simulink model "lab_single_phse_inv_1"  (R2019a)
settings: Solver=VariableStepAuto  StartTime=0.0  StopTime=0.1  RelTol=1e-3
libraries: powerlib x12, simulink x1
settings Model: Creator=Manish  LastModifiedBy=Manish

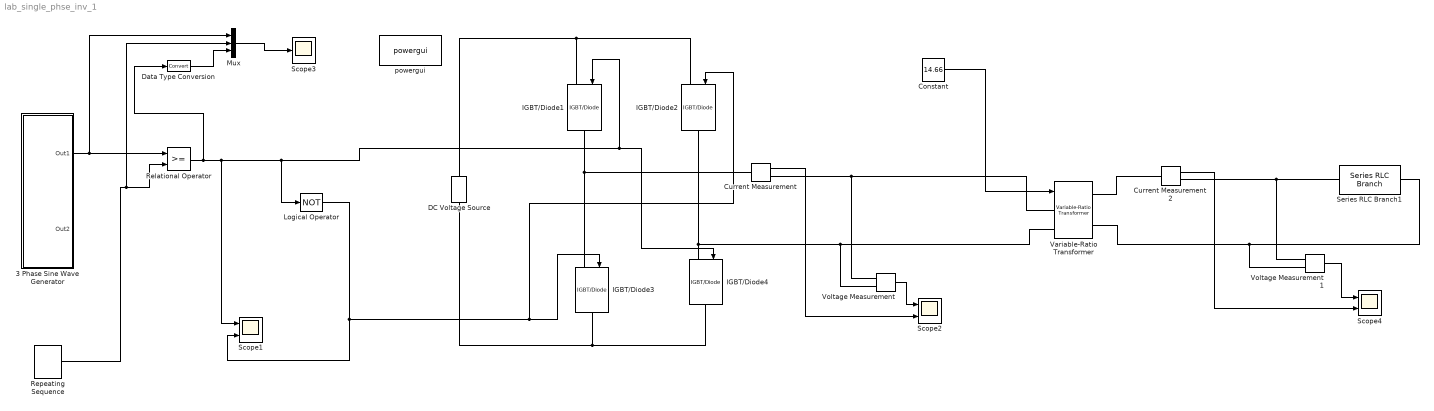
== system lab_single_phse_inv_1 ==
  3 Phase Sine Wave Generator : Subsystem
  Constant : Constant  Value=14.66
  Current Measurement : powerlib/Measurements/Current Measurement  PhasorSimulation=off  OutputType=Complex  PSBequivalent=0
  Current Measurement2 : powerlib/Measurements/Current Measurement  PhasorSimulation=off  OutputType=Complex  PSBequivalent=0
  DC Voltage Source : powerlib/Electrical Sources/DC Voltage Source  Amplitude=24  Measurements=None
  Data Type Conversion : DataTypeConversion
  IGBT/Diode{1..4} (4 alike) : powerlib/Power Electronics/IGBT//Diode  Ron=1e-3  Rs=1e5  Cs=inf  Measurements=off
  Logical Operator : Logic  Operator=NOT  AllPortsSameDT=off  OutDataTypeStr=boolean
  Mux : Mux  Inputs=3
  Relational Operator : RelationalOperator  RndMeth=Nearest
  Repeating Sequence : simulink/Sources/Repeating Sequence  rep_seq_t=[0 0.25 0.5 0.75 1]/1000  rep_seq_y=[0 1 0 -1 0]
  Scope1 : Scope  NumInputPorts=2
  Scope2 : Scope  NumInputPorts=2
  Scope3 : Scope
  Scope4 : Scope  NumInputPorts=2
  Series RLC Branch1 : powerlib/Elements/Series RLC Branch  LConnTagsString=__new0  RConnTagsString=__new0  BranchType=RL  Resistance=10  Inductance=10e-3  SetiL0=off  InitialCurrent=0  Capacitance=1e-6  Setx0=off  InitialVoltage=0  Measurements=None
  Variable-Ratio Transformer : powerlib/Elements/Variable-Ratio Transformer
      settings: SourceProductBaseCode=PS
  Voltage Measurement : powerlib/Measurements/Voltage Measurement  PhasorSimulation=off  OutputType=Complex  PSBequivalent=0
  Voltage Measurement1 : powerlib/Measurements/Voltage Measurement  PhasorSimulation=off  OutputType=Complex  PSBequivalent=0
  powergui : powerlib/powergui  Priority=1  SimulationMode=Discrete  SampleTime=1e-6  frequency=60  Iterations=50  frequencyindice=0  Pbase=100e6  ErrMax=1e-4  UnitsV=kV  UnitsW=MW  buscounter=0  FunctionMessages=off  echomessages=off  EnableUseOfTLC=off  CurrentSourceSwitches=off  DisableSnubberDevices=off  DisableRonSwitches=off  DisableVfSwitches=off  DisplayEquations=off  AutomaticDiscreteSolvers=off  SolverType=Tustin/Backward Euler (TBE)  Interpol=off  ExternalGateDelay=off  methode=off  Ts=100  x0status=blocks  SPID=on  SwTol=0  HookPort=off  NonlinearTolerance=1e-4  nMaxIteration=100  ContinueOnMaxIteration=off  RestoreLinks=warning  ResistiveCurrentMeasurement=off  Frange=[0:2:500]  Ylog=off  Xlog=on  ShowGrid=off  save=off  variable=ZData  structure=voltage_current  ZoomFFT=off  StartTime=0.0  cycles=2  DisplayStyle=2  fundamental=50  FreqAxis=off  MaxFrequency=20000  frequencyindicesteady=1  RmsSteady=1  display=off
  wires:
  3 Phase Sine Wave Generator/1(Out1) -> Mux/1, Relational Operator/1
  Repeating Sequence/1 -> Mux/2, Relational Operator/2
  Relational Operator/1 -> Data Type Conversion/1, IGBT/Diode4/1, IGBT/Diode1/1, Logical Operator/1, Scope1/1
  Logical Operator/1 -> IGBT/Diode3/1, IGBT/Diode2/1, Scope1/2
  Voltage Measurement/1 -> Scope2/1
  Current Measurement/1 -> Scope2/2
  Voltage Measurement1/1 -> Scope4/1
  Current Measurement2/1 -> Scope4/2
  Mux/1 -> Scope3/1
  Data Type Conversion/1 -> Mux/3
  Constant/1 -> Variable-Ratio Transformer/1
  connections:
  DC Voltage Source/RConn1 -- IGBT/Diode2/LConn1 -- IGBT/Diode1/LConn1
  DC Voltage Source/LConn1 -- IGBT/Diode4/RConn1 -- IGBT/Diode3/RConn1
  Current Measurement/LConn1 -- IGBT/Diode3/LConn1 -- IGBT/Diode1/RConn1
  Voltage Measurement/LConn1 -- Variable-Ratio Transformer/LConn1 -- Current Measurement/RConn1
  Voltage Measurement/LConn2 -- Variable-Ratio Transformer/LConn2 -- IGBT/Diode2/RConn1 -- IGBT/Diode4/LConn1
  Current Measurement2/RConn1 -- Voltage Measurement1/LConn1 -- Series RLC Branch1/LConn1
  Current Measurement2/LConn1 -- Variable-Ratio Transformer/RConn1
  Variable-Ratio Transformer/RConn2 -- Series RLC Branch1/RConn1 -- Voltage Measurement1/LConn2

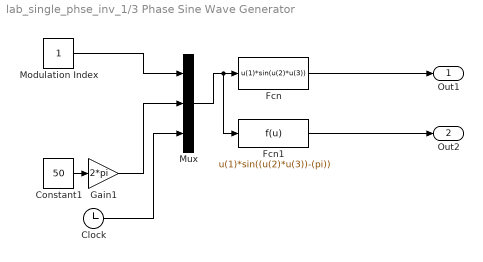
== system lab_single_phse_inv_1/3 Phase Sine Wave Generator ==
  Clock : Clock
      settings: Decimation=100
  Constant1 : Constant  Value=50
  Fcn : Fcn  Expr=u(1)*sin(u(2)*u(3))
  Fcn1 : Fcn  Expr=u(1)*sin((u(2)*u(3))-(pi))
  Gain1 : Gain  Gain=2*pi
  Modulation Index : Constant
  Mux : Mux  Inputs=3
  Out1 : Outport
  Out2 : Outport  Port=2
  wires:
  Gain1/1 -> Mux/2
  Mux/1 -> Fcn/1, Fcn1/1
  Fcn/1 -> Out1/1
  Fcn1/1 -> Out2/1
  Modulation Index/1 -> Mux/1
  Clock/1 -> Mux/3
  Constant1/1 -> Gain1/1
